simulink model "reservoirs_ardc"  (R2024b)
settings: Solver=ode45  StartTime=0.0  StopTime=200  MaxStep=0.05  RelTol=1e-3
libraries: simulink x2, slctrl_adaptive x1
settings Model: Creator=dsychel  LastModifiedBy=zv53855

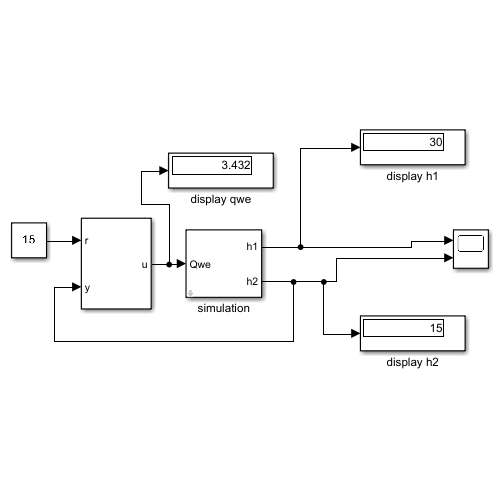
[thumbnail: Simulink's stored preview of the top-level diagram]
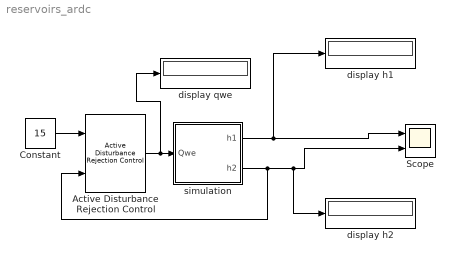
== system reservoirs_ardc ==
  Active Disturbance Rejection Control : slctrl_adaptive/Active Disturbance Rejection Control  time_domain=discrete-time  Ts=0.01  model_type=first-order  b0=1  wc=0.1  wo=2  x0=0  ulim_checkbox=off  umax=inf  umin=-inf  xhat_checkbox=off
      settings: LibrarySourceBlock=slctrlblks/Adaptive Control/Active Disturbance Rejection Control
  Constant : Constant  Value=15
  Scope : Scope  NumInputPorts=2
  display h1 : Display
  display h2 : Display
  display qwe : Display
  simulation : Subsystem  mask{h1_0=4, h2_0=2, S1=1, S2=2, Swy1=0.2, Swy2=0.2, phi1=1, phi2=1, g=9.81, Qwe=5.374}
      mask prompts: h1_0 "liquid level 1 init"; h2_0 "liquid level 2 init"; S1 "cross section reservoir 1"; S2 "cross section reservoir 2"; Swy1 "cross section outflow 1"; Swy2 "cross section outflow 2"; phi1 "coef 1"; phi2 "coef 2"; Qwe "liquid tributary"
  wires:
  simulation/2(h2) -> Active Disturbance Rejection Control/2, display h2/1, Scope/2
  simulation/1(h1) -> display h1/1, Scope/1
  Active Disturbance Rejection Control/1 -> display qwe/1, simulation/1(Qwe)
  Constant/1 -> Active Disturbance Rejection Control/1

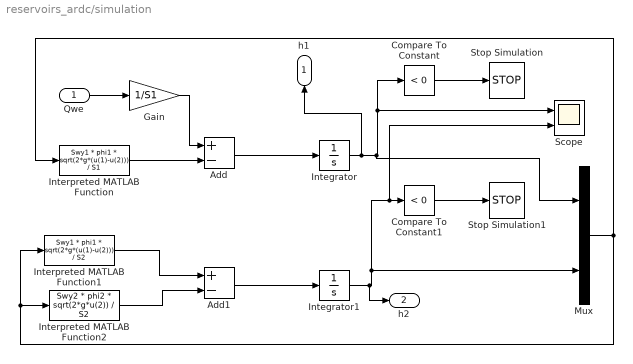
== system reservoirs_ardc/simulation ==
  Qwe : Inport
  Add : Sum  Inputs=+-
  Add1 : Sum  Inputs=+-
  Compare To Constant : simulink/Logic and Bit Operations/Compare To Constant  relop=<  const=0  OutDataTypeStr=boolean
  Compare To Constant1 : simulink/Logic and Bit Operations/Compare To Constant  relop=<  const=0  OutDataTypeStr=boolean
  Gain : Gain  Gain=1/S1
  Integrator : Integrator  InitialCondition=h1_0
  Integrator1 : Integrator  InitialCondition=h2_0
  Interpreted MATLAB Function : MATLABFcn  MATLABFcn=Swy1 * phi1 * sqrt(2*g*(u(1)-u(2))) / S1
  Interpreted MATLAB Function1 : MATLABFcn  MATLABFcn=Swy1 * phi1 * sqrt(2*g*(u(1)-u(2))) / S2
  Interpreted MATLAB Function2 : MATLABFcn  MATLABFcn=Swy2 * phi2 * sqrt(2*g*u(2)) / S2
  Mux : Mux  Inputs=2
  Scope : Scope  NumInputPorts=2
  Stop Simulation : Stop
  Stop Simulation1 : Stop
  h1 : Outport
  h2 : Outport  Port=2
  wires:
  Compare To Constant/1 -> Stop Simulation/1
  Add/1 -> Integrator/1
  Integrator/1 -> h1/1, Mux/1, Scope/1, Compare To Constant/1
  Gain/1 -> Add/1
  Interpreted MATLAB Function/1 -> Add/2
  Compare To Constant1/1 -> Stop Simulation1/1
  Integrator1/1 -> h2/1, Mux/2, Scope/2, Compare To Constant1/1
  Add1/1 -> Integrator1/1
  Interpreted MATLAB Function1/1 -> Add1/1
  Interpreted MATLAB Function2/1 -> Add1/2
  Mux/1 -> Interpreted MATLAB Function2/1, Interpreted MATLAB Function1/1, Interpreted MATLAB Function/1
  Qwe/1 -> Gain/1
